simulink model "sg_IK"  (R2021b)
settings: Solver=ode4  StartTime=0.0  StopTime=10  FixedStep=Ts  RelTol=1e-3  EnableMultiTasking=on
model workspace (MAT data in the model file):
  BList = [0 0 -1 0 -2.61918 0 0 1 0 1.41 0 -2.26918 ... (30 elements, 6x5)]
  M = [1 0 0 0 0 1 0 0 0 0 1 0 ... (16 elements, 4x4)]
  Manual_State_Switch = 0
  Operation_Mode = 2
  SList = [0 0 -1 0 0 0 0 1 0 -0.83 0 0.35 ... (30 elements, 6x5)]
  State_Mode_Selector = 2
  Traj_method = 1
  Winch_EnableHeaveComp = 0
  Winch_NewCmd = 0
  Winch_PosRef = 10
  controlMode = 2
  new_command_traj = 0
  v_max = 0
  x_coordinate_traj = 0
  y_coordinate_traj = 0
  z_coordinate_traj = 0
values from neighbouring files (symbols this model uses):
  Ts = 1e-3    (= 0.001)    [sg_IK_build.m]    (also in sg_IK_startup.m)
libraries: slpidlib x5, slrealtimeutilitieslib x3, slrealtimeiplib x3, dspfdesign x1
(part 2 of 2)

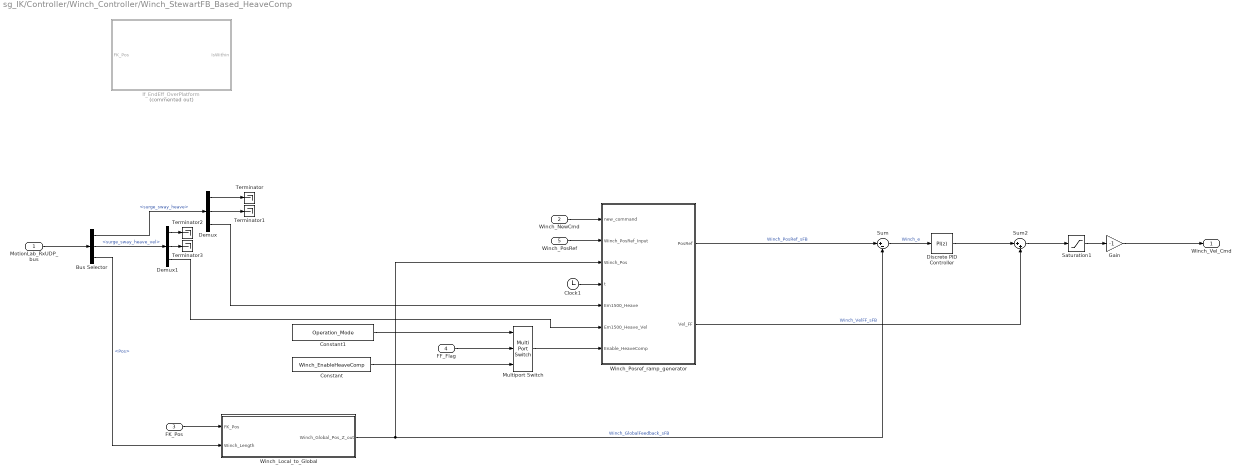
== system sg_IK/Controller/Winch_Controller/Winch_StewartFB_Based_HeaveComp ==
  MotionLab_RxUDP_bus : Inport
  Winch_NewCmd : Inport  Port=2
  FK_Pos : Inport  Port=3
  FF_Flag : Inport  Port=4
  Winch_PosRef : Inport  Port=5
  Bus Selector : BusSelector  OutputSignals=Em1500.surge_sway_heave,Em1500.surge_sway_heave_vel,Comau_winch.Pos
  Clock1 : Clock
  Constant : Constant  Value=Winch_EnableHeaveComp
  Constant1 : Constant  Value=Operation_Mode
  Demux : Demux  Outputs=3
  Demux1 : Demux  Outputs=3
  Discrete PID Controller : slpidlib/PID Controller  Controller=PI  Form=Parallel  TimeDomain=Discrete-time  UseExternalTs=off  SampleTime=Ts  IntegratorMethod=Forward Euler  FilterMethod=Forward Euler  ControllerParametersSource=internal  P=2  I=0.09  D=0  UseFilter=on  N=100  TunerSelectOption=Transfer Function Based (PID Tuner App)  InitialConditionSource=internal  InitialConditionForIntegrator=0  InitialConditionForFilter=0  DifferentiatorICPrevScaledInput=0  ExternalReset=none  TrackingMode=off  Kt=1  LimitOutput=off  SatLimitsSource=internal  UpperSaturationLimit=inf  LowerSaturationLimit=-inf  LinearizeAsGain=off  AntiWindupMode=none  Kb=1  POutMin=[]  POutMax=[]  IOutMin=[]  IOutMax=[]  DOutMin=[]  DOutMax=[]  NOutMin=[]  NOutMax=[]  SumOutMin=[]  SumOutMax=[]  SaturationOutMin=[]  SaturationOutMax=[]  PParamMin=[]  PParamMax=[]  IParamMin=[]  IParamMax=[]  DParamMin=[]  DParamMax=[]  NParamMin=[]  NParamMax=[]  KbParamMin=[]  KbParamMax=[]  KtParamMin=[]  KtParamMax=[]  KbOutMin=[]  KbOutMax=[]  KtOutMin=[]  KtOutMax=[]  IntegratorOutMin=[]  IntegratorOutMax=[]  FilterOutMin=[]  FilterOutMax=[]  SumI1OutMin=[]  SumI1OutMax=[]  SumI2OutMin=[]  SumI2OutMax=[]  SumI3OutMin=[]  SumI3OutMax=[]  SumI4OutMin=[]  SumI4OutMax=[]  SumDOutMin=[]  SumDOutMax=[]  DifferentiatorOutMin=[]  DifferentiatorOutMax=[]  FilterDiffOutCoefMin=[]  FilterDiffOutCoefMax=[]  ReciprocalOutMin=[]  ReciprocalOutMax=[]  SumDenOutMin=[]  SumDenOutMax=[]  SumNumOutMin=[]  SumNumOutMax=[]  DivideOutMin=[]  DivideOutMax=[]  UdiffTsProdOutMin=[]  UdiffTsProdOutMax=[]  NTsProdOutMin=[]  NTsProdOutMax=[]  UintegralTsProdOutMin=[]  UintegralTsProdOutMax=[]  UngainTsProdOutMin=[]  UngainTsProdOutMax=[]  FilterDenConstantOutDataTypeStr=Inherit: Inherit via back propagation  FilterDenConstantOutMin=[]  FilterDenConstantOutMax=[]  PCopyOutDataTypeStr=Inherit: Inherit via back propagation  PCopyOutMin=[]  PCopyOutMax=[]  NCopyOutDataTypeStr=Inherit: Inherit via back propagation  NCopyOutMin=[]  NCopyOutMax=[]  IntegratorContinuousStateAttributes=''  IntegratorStateMustResolveToSignalObject=off  IntegratorRTWStateStorageClass=Auto  FilterContinuousStateAttributes=''  FilterStateMustResolveToSignalObject=off  FilterRTWStateStorageClass=Auto  ParallelPVariant=InternalParameters  IdealPVariant=Disabled  IVariant=InternalParameters  DVariant=Disabled  IntegratorVariant=Discrete  SatVariant=Disabled  AWVariant=Passthrough  PCopyVariant=Disabled  TRVariant=Disabled  FdbkBlocksVariant=Forward  IdealPFdbkVariant=Disabled  SatFdbkVariant=Disabled  DerivativeFilterVariant=Disabled  NVariant=Disabled  NCopyVariant=Disabled_SignalSpec  FilterICVariant=Disabled  IntegratorICVariant=InternalICs  ExternalResetVariant=Disabled  TRSumVariant=Passthrough  SumFdbkVariant=Disabled  SumVariant=Sum_PI  TsampFilterVariant=InternalTs  TsampNgainVariant=Passthrough  TsampIntegralVariant=Passthrough  ExternalSaturationOutDataTypeStr=Inherit: Same as second input
  Gain : Gain  Gain=-1
  If_EndEff_OverPlatform : MATLAB Function  Commented=on  TreatAsAtomicUnit=on
  Multiport Switch : MultiPortSwitch  Inputs=2
  Saturation1 : Saturate  UpperLimit=0.2  LowerLimit=-0.2
  Sum : Sum  Inputs=|+-
  Sum2 : Sum  Inputs=|++
  Terminator{,1..3} (4 alike) : Terminator
  Winch_Local_to_Global : MATLAB Function  TreatAsAtomicUnit=on
  Winch_Posref_ramp_generator : MATLAB Function  TreatAsAtomicUnit=on
  Winch_Vel_Cmd : Outport
  wires:
  Constant/1 -> Multiport Switch/3
  Constant1/1 -> Multiport Switch/1
  Multiport Switch/1 -> Winch_Posref_ramp_generator/7(Enable_HeaveComp)
  Clock1/1 -> Winch_Posref_ramp_generator/4(t)
  Winch_NewCmd/1 -> Winch_Posref_ramp_generator/1(new_command)
  Winch_PosRef/1 -> Winch_Posref_ramp_generator/2(Winch_PosRef_Input)
  FF_Flag/1 -> Multiport Switch/2
  Discrete PID Controller/1 -> Sum2/1
  Winch_Posref_ramp_generator/1(PosRef) -> Sum/1  "Winch_PosRef_sFB"
  Winch_Posref_ramp_generator/2(Vel_FF) -> Sum2/2  "Winch_VelFF_sFB"
  Saturation1/1 -> Gain/1
  Sum/1 -> Discrete PID Controller/1  "Winch_e"
  Sum2/1 -> Saturation1/1
  FK_Pos/1 -> Winch_Local_to_Global/1(FK_Pos)
  MotionLab_RxUDP_bus/1 -> Bus Selector/1
  Bus Selector/3 -> Winch_Local_to_Global/2(Winch_Length)  "<Pos>"
  Winch_Local_to_Global/1(Winch_Global_Pos_Z_out) -> Winch_Posref_ramp_generator/3(Winch_Pos), Sum/2  "Winch_GlobalFeedback_sFB"
  Bus Selector/1 -> Demux/1  "<surge_sway_heave>"
  Demux/1 -> Terminator/1
  Demux/2 -> Terminator1/1
  Demux/3 -> Winch_Posref_ramp_generator/5(Em1500_Heave)
  Bus Selector/2 -> Demux1/1  "<surge_sway_heave_vel>"
  Demux1/1 -> Terminator2/1
  Demux1/2 -> Terminator3/1
  Demux1/3 -> Winch_Posref_ramp_generator/6(Em1500_Heave_Vel)
  Gain/1 -> Winch_Vel_Cmd/1

== matlab function sg_IK/Controller/State Machine and Operation mode selecotr/Winch_Local_to_Global ==
  data: FK_Pos input; Winch_Global_Pos_Z output; Winch_Length input
function Winch_Global_Pos_Z = Winch_Global_Pos(FK_Pos, Winch_Length)
    %constant found from calibrating winch moving it to same height as
    %ball
    vertical_distance = Winch_Length - 0.202; 
    Winch_Global_Pos_Z = FK_Pos(3) - vertical_distance;
end

== matlab function sg_IK/Controller/Winch_Controller/Winch_StewartFB_Based_HeaveComp/Winch_Local_to_Global ==
  data: FK_Pos input; Winch_Global_Pos_Z_out output; Winch_Length input
function Winch_Global_Pos_Z_out = Winch_Global_Pos( FK_Pos, Winch_Length)

vertical_distance = Winch_Length - 0.202; 

Winch_Global_Pos_Z_out = FK_Pos(3) - vertical_distance;



end

== matlab function sg_IK/Controller/State Machine and Operation mode selecotr/is_Em8000_settled ==
  data: Em8000_translation input; Em8000_settled_flag output
function Em8000_settled_flag = settled_fnc(Em8000_translation)
Em8000_heave = Em8000_translation(3);

%Flag for if platform is in settled position
%More better handling would be a direct feedback from the Em1500 IPC what operation mode the platform is in
if Em8000_heave >= 0.99 && Em8000_heave <= 1.01 %Em1500 platform is in settled mode
    Em8000_settled_flag = true;
else
    Em8000_settled_flag = false;
end

== stateflow chart sg_IK/Controller/State Machine and Operation mode selecotr/Chart ==
  state Manual_State_Switch_Mode
    state Go_home
      entry:
      if Em8000_settled_flag && ~Em8000_comp_offset_flag
      Em8000_settled_offset = 1;
      elseif Em8000_comp_offset_flag
      Em8000_settled_offset = 0.65;
      else
      Em8000_settled_offset = 0;
      end
      X_home = -0.9;
      Y_home = -1.3;
      Z_home = 5.9 - Em8000_settled_offset;
      Traj_points_XYZ = [FK_Pos(1), X_home, FK_Pos(2), Y_home, FK_Pos(3), Z_home];
      Traj_method = 2;
      v_max = 0.1;
      new_command = new_command + 1;
      Winch_PosRef = 10; %JUST MOVE UP, MAKE MORE ROBUST LATER
      Winch_Mode_selector = 1;
      FF_Flag = 0;
    state Stay_in_current_position
      entry:
      % Set the values for the variables
      Traj_points_XYZ = [FK_Pos(1), FK_Pos(1), FK_Pos(2), FK_Pos(2), FK_Pos(3), FK_Pos(3)];
      Traj_method = 1;
      v_max = 0;
      new_command = new_command + 1;
      FF_Flag = 0;
      Winch_PosRef = 10; %Just move up to endstop
      Winch_Mode_selector = 1; %REMOVE LATER
    state Move_to_above_platform_PickUp
      %Move above platform to initiate hooking and pick up of payload
      entry:
      if Em8000_settled_flag && ~Em8000_comp_offset_flag
      Em8000_settled_offset = 1;
      elseif Em8000_comp_offset_flag
      Em8000_settled_offset = 0.65;
      else
      Em8000_settled_offset = 0;
      end
      X_Platform = 0.42;
      Y_Platform = -1.57;
      Z_Platform = 5.62 - Em8000_settled_offset;
      Traj_points_XYZ = [FK_Pos(1), X_Platform, FK_Pos(2), Y_Platform, FK_Pos(3), Z_Platform];
      Traj_method = 2;
      v_max = 0.12;
      new_command = new_command + 1;
      %move winch
      Winch_Mode_selector = 1;
      Winch_PosRef = 3.2;
      %Winch_NewCmd = Winch_NewCmd + 1;
      FF_Flag = 0;
      during:
      Winch_PosRef = 3.2;
    state Hook_Ball
      state Ball_In_Frame
        %If ball not in frame wait over platform
        entry:
        if bBall_InFrame
        Sub_stage_switch = 1;
        else
        Sub_stage_switch = 0;
        Traj_points_XYZ = [FK_Pos(1), FK_Pos(1), FK_Pos(2), FK_Pos(2), FK_Pos(3), FK_Pos(3)];
        v_max = 0;
        new_command = new_command + 1;
        end
        during:
        if bBall_InFrame
        Sub_stage_switch = 1;
        end
      state Move_Close_To_Ball
        entry:
        Z_Offset = 0.15;
        r_Offset = 0.15;  % Radius offset to ball
        % Compute the approach vector in xy plane
        delta_xy = FK_Pos(1:2) - Ball_Pos(1:2);
        norm_delta = norm(delta_xy);
        if norm_delta < 1e-6
        Target_Pos_X = FK_Pos(1);
        Target_Pos_Y = FK_Pos(2);
        v_max = 0;
        else
        unit_delta = delta_xy / norm_delta;
        Target_Pos_X = Ball_Pos(1) + r_Offset * unit_delta(1);
        Target_Pos_Y = Ball_Pos(2) + r_Offset * unit_delta(2);
        v_max = 0.05;
        end
        %Target_Pos_Z = Ball_Pos(3) + Winch_PosRef + Z_Offset;
        Traj_points_XYZ = [FK_Pos(1), Target_Pos_X, FK_Pos(2), Target_Pos_Y, FK_Pos(3), FK_Pos(3)];
        Traj_method = 2;
        new_command = new_command + 1;
        Winch_PosRef = Ball_Pos(3) - Z_Offset;
        FF_Flag = 1;
        during:
        Winch_PosRef = Ball_Pos(3) - Z_Offset;
        if ~traj_running
        Sub_stage_switch = 2;
        else
        Sub_stage_switch = 1;
        end
      state Move_in_to_ball
        entry:
        Z_Offset = 0.07;
        %Winch_neutral_length = Winch_PosRef;
        Traj_points_XYZ = [FK_Pos(1), Ball_Pos(1), FK_Pos(2), Ball_Pos(2)+0.04, FK_Pos(3), FK_Pos(3)];
        Traj_method = 2;
        v_max = 0.02;
        new_command = new_command + 1;
        Winch_PosRef = Ball_Pos(3);
        FF_Flag = 1;
        during:
        %CB_Absdelta_X = abs(Ball_Pos(1) - Claw_Pos(1));
        %CB_Absdelta_Y = abs(Ball_Pos(2) - Claw_Pos(2));
        Winch_PosRef = Ball_Pos(3) - Z_Offset;
        if ~traj_running
        Sub_stage_switch = 3;
        else
        Sub_stage_switch = 2;
        end
      state Lift_Up
        entry:
        FF_Flag = 0;
        Winch_PosRef = 10;
      (default) -> Manual_State_Switch_Mode.Hook_Ball.Ball_In_Frame
      Manual_State_Switch_Mode.Hook_Ball.Ball_In_Frame -> Manual_State_Switch_Mode.Hook_Ball.Move_Close_To_Ball : [Sub_stage_switch == 1]
      Manual_State_Switch_Mode.Hook_Ball.Move_Close_To_Ball -> Manual_State_Switch_Mode.Hook_Ball.Move_in_to_ball : [Sub_stage_switch == 2 && after(1, sec)]
      Manual_State_Switch_Mode.Hook_Ball.Move_in_to_ball -> Lift_Up : [Sub_stage_switch == 3]
    state Lower_payload_Onto_platform
      state Move_above_platform_While_lowering_payload
        %Move above platform and start moving winch down to stewart platform netrual position to follow
        %And follow heave motion
        entry:
        if Em8000_settled_flag && ~Em8000_comp_offset_flag
        Em8000_settled_offset = 1;
        elseif Em8000_comp_offset_flag
        Em8000_settled_offset = 0.65;
        else
        Em8000_settled_offset = 0;
        end
        Sub_stage_switch2 = 0;
        X_Platform = 0.41;
        Y_Platform = -1.34;
        Z_Platform = 5.67 - Em8000_settled_offset;
        Traj_points_XYZ = [FK_Pos(1), X_Platform, FK_Pos(2), Y_Platform, FK_Pos(3), Z_Platform];
        Traj_method = 2;
        v_max = 0.12;
        new_command = new_command + 1;
        %move winch
        Winch_Mode_selector = 2;
        Winch_PosRef = 2.6;
        Winch_NewCmd = Winch_NewCmd + 1;
        FF_Flag = 1;
        during:
        if ~traj_running
        Sub_stage_switch2 = 1;
        end
      state Lower_winch_To_unhook
        entry:
        Winch_PosRef = 2.6;
        Winch_NewCmd = Winch_NewCmd + 1;
      state Move_to_side_unhook
        entry:
        if Em8000_settled_flag && ~Em8000_comp_offset_flag
        Em8000_settled_offset = 1;
        elseif Em8000_comp_offset_flag
        Em8000_settled_offset = 0.65;
        else
        Em8000_settled_offset = 0;
        end
        X_Unhook = 0;
        Y_Unhook = -1.62;
        Z_Unhook = 5.62 - Em8000_settled_offset;
        Traj_points_XYZ = [FK_Pos(1), X_Unhook, FK_Pos(2), Y_Unhook, FK_Pos(3), Z_Unhook];
        Traj_method = 2;
        v_max = 0.07;
        new_command = new_command + 1;
        %move winch
        Winch_PosRef = 2.6;
        Winch_NewCmd = Winch_NewCmd + 1;
        FF_Flag = 1;
      (default) -> Manual_State_Switch_Mode.Lower_payload_Onto_platform.Move_above_platform_While_lowering_payload
      Manual_State_Switch_Mode.Lower_payload_Onto_platform.Move_above_platform_While_lowering_payload -> Manual_State_Switch_Mode.Lower_payload_Onto_platform.Lower_winch_To_unhook : [Sub_stage_switch2 == 1 && after(3, sec)]
      Manual_State_Switch_Mode.Lower_payload_Onto_platform.Lower_winch_To_unhook -> Manual_State_Switch_Mode.Lower_payload_Onto_platform.Move_to_side_unhook : [after(7, sec)]
    (default) -> Stay_in_current_position
    Manual_State_Switch_Mode.Lower_payload_Onto_platform -> Manual_State_Switch_Mode.Go_home [order 1] : [Switch == 1]
    Manual_State_Switch_Mode.Go_home -> Manual_State_Switch_Mode.Lower_payload_Onto_platform [order 3] : [Switch == 4]
    Stay_in_current_position -> Manual_State_Switch_Mode.Go_home [order 1] : [Switch == 1]
    Manual_State_Switch_Mode.Hook_Ball -> Manual_State_Switch_Mode.Go_home [order 2] : [Switch == 1]
    Manual_State_Switch_Mode.Go_home -> Stay_in_current_position [order 1] : [Switch == 0]
    Manual_State_Switch_Mode.Lower_payload_Onto_platform -> Stay_in_current_position [order 2] : [Switch == 0]
    Manual_State_Switch_Mode.Hook_Ball -> Stay_in_current_position [order 3] : [Switch == 0]
    Manual_State_Switch_Mode.Move_to_above_platform_PickUp -> Stay_in_current_position [order 1] : [Switch == 0]
    Stay_in_current_position -> Manual_State_Switch_Mode.Move_to_above_platform_PickUp [order 2] : [Switch == 2]
    Manual_State_Switch_Mode.Move_to_above_platform_PickUp -> Manual_State_Switch_Mode.Go_home [order 2] : [Switch == 1]
    Manual_State_Switch_Mode.Go_home -> Manual_State_Switch_Mode.Move_to_above_platform_PickUp [order 2] : [Switch == 2]
    Manual_State_Switch_Mode.Move_to_above_platform_PickUp -> Manual_State_Switch_Mode.Hook_Ball [order 3] : [Switch == 3]
    Manual_State_Switch_Mode.Hook_Ball -> Manual_State_Switch_Mode.Move_to_above_platform_PickUp [order 1] : [Switch==2]
  state Mode_selector_state
    entry:
    %Entry state to choose between manual state switch mode or Autonomous mode
    if State_Mode_Selector == 1 %Autonomous mode
    Hook_state_switch = 1;
    Mode = 1;
    elseif  State_Mode_Selector == 2 %Manual state switch mode
    Mode = 2;
    else %Default to Manual state switch mode
    Mode = 2;
    end
  state Autonomous_Operation_Mode
    state Go_home
      entry:
      AutoSwitch = 0;
      if Em8000_settled_flag && ~Em8000_comp_offset_flag
      Em8000_settled_offset = 1;
      elseif Em8000_comp_offset_flag
      Em8000_settled_offset = 0.65;
      else
      Em8000_settled_offset = 0;
      end
      X_home = -0.9;
      Y_home = -1.3;
      Z_home = 5.9 - Em8000_settled_offset;
      Traj_points_XYZ = [FK_Pos(1), X_home, FK_Pos(2), Y_home, FK_Pos(3), Z_home];
      Traj_method = 2;
      v_max = 0.1;
      new_command = new_command + 1;
      Winch_PosRef = 10; %JUST MOVE UP, MAKE MORE ROBUST LATER
      Winch_Mode_selector = 1;
      FF_Flag = 0;
      during:
      if ~traj_running
      if Hook_state_switch == 1
      AutoSwitch = 1; %Hook payload
      else
      AutoSwitch = 2; %Lower payload
      end
      else
      AutoSwitch = 0; %Stay in current state until traj to home complete
      end
    state Hook_Ball
      state Move_to_above_platform_PickUp
        %Move above platform to initiate hooking and pick up of payload
        entry:
        if Em8000_settled_flag && ~Em8000_comp_offset_flag
        Em8000_settled_offset = 1;
        elseif Em8000_comp_offset_flag
        Em8000_settled_offset = 0.65;
        else
        Em8000_settled_offset = 0;
        end
        X_Platform = 0.42;
        Y_Platform = -1.57;
        Z_Platform = 5.62 - Em8000_settled_offset;
        Traj_points_XYZ = [FK_Pos(1), X_Platform, FK_Pos(2), Y_Platform, FK_Pos(3), Z_Platform];
        Traj_method = 2;
        v_max = 0.16;
        new_command = new_command + 1;
        %move winch
        Winch_Mode_selector = 1;
        Winch_PosRef = 3.15;
        %Winch_NewCmd = Winch_NewCmd + 1;
        FF_Flag = 1;
        during:
        Winch_PosRef = 3.15;
        if ~traj_running
        Sub_stage_switch = 1;
        end
      state Ball_In_Frame
        %If ball not in frame wait over platform
        entry:
        if bBall_InFrame
        Sub_stage_switch = 1;
        else
        Sub_stage_switch = 0;
        Traj_points_XYZ = [FK_Pos(1), FK_Pos(1), FK_Pos(2), FK_Pos(2), FK_Pos(3), FK_Pos(3)];
        v_max = 0;
        new_command = new_command + 1;
        end
        during:
        if bBall_InFrame
        Sub_stage_switch = 2;
        else
        Sub_stage_switch = 1;
        end
      state Move_Close_To_Ball
        entry:
        Z_Offset = 0.15;
        r_Offset = 0.15;  % Radius offset to ball
        % Compute the approach vector in xy plane
        delta_xy = FK_Pos(1:2) - Ball_Pos(1:2);
        norm_delta = norm(delta_xy);
        if norm_delta < 1e-6
        Target_Pos_X = FK_Pos(1);
        Target_Pos_Y = FK_Pos(2);
        v_max = 0;
        else
        unit_delta = delta_xy / norm_delta;
        Target_Pos_X = Ball_Pos(1) + r_Offset * unit_delta(1);
        Target_Pos_Y = Ball_Pos(2) + r_Offset * unit_delta(2);
        v_max = 0.02;
        end
        %Target_Pos_Z = Ball_Pos(3) + Winch_PosRef + Z_Offset;
        Traj_points_XYZ = [FK_Pos(1), Target_Pos_X, FK_Pos(2), Target_Pos_Y, FK_Pos(3), FK_Pos(3)];
        Traj_method = 2;
        new_command = new_command + 1;
        Winch_PosRef = Ball_Pos(3) - Z_Offset;
        FF_Flag = 1;
        during:
        Winch_PosRef = Ball_Pos(3) - Z_Offset;
        if ~traj_running
        Sub_stage_switch = 3;
        else
        Sub_stage_switch = 2;
        end
      state Move_in_to_ball
        entry:
        Z_Offset = 0.07;
        %Winch_neutral_length = Winch_PosRef;
        Traj_points_XYZ = [FK_Pos(1), Ball_Pos(1), FK_Pos(2), Ball_Pos(2)+0.06, FK_Pos(3), FK_Pos(3)];
        Traj_method = 2;
        v_max = 0.02;
        new_command = new_command + 1;
        Winch_PosRef = Ball_Pos(3);
        FF_Flag = 1;
        during:
        %CB_Absdelta_X = abs(Ball_Pos(1) - Claw_Pos(1));
        %CB_Absdelta_Y = abs(Ball_Pos(2) - Claw_Pos(2));
        Winch_PosRef = Ball_Pos(3) - Z_Offset;
        if ~traj_running
        AutoSwitch = 0;
        else
        Sub_stage_switch = 2;
        end
        exit:
        Sub_stage_switch = 0;
        Hook_state_switch = 0; %Payload was picked up mark next exit from Go_to_home to lower payload
      (default) -> Autonomous_Operation_Mode.Hook_Ball.Move_to_above_platform_PickUp
      Autonomous_Operation_Mode.Hook_Ball.Move_to_above_platform_PickUp -> Autonomous_Operation_Mode.Hook_Ball.Ball_In_Frame : [Sub_stage_switch == 1 && after(1, sec)]
      Autonomous_Operation_Mode.Hook_Ball.Ball_In_Frame -> Autonomous_Operation_Mode.Hook_Ball.Move_Close_To_Ball : [Sub_stage_switch == 2]
      Autonomous_Operation_Mode.Hook_Ball.Move_Close_To_Ball -> Autonomous_Operation_Mode.Hook_Ball.Move_in_to_ball : [Sub_stage_switch == 3 && after(0.5, sec)]
    state Lower_payload_Onto_platform
      state Move_above_platform_While_lowering_payload
        %Move above platform and start moving winch down to stewart platform netrual position to follow
        %And follow heave motion
        entry:
        if Em8000_settled_flag && ~Em8000_comp_offset_flag
        Em8000_settled_offset = 1;
        elseif Em8000_comp_offset_flag
        Em8000_settled_offset = 0.65;
        else
        Em8000_settled_offset = 0;
        end
        Sub_stage_switch2 = 0;
        X_Platform = 0.41;
        Y_Platform = -1.34;
        Z_Platform = 5.67 - Em8000_settled_offset;
        Traj_points_XYZ = [FK_Pos(1), X_Platform, FK_Pos(2), Y_Platform, FK_Pos(3), Z_Platform];
        Traj_method = 2;
        v_max = 0.16;
        new_command = new_command + 1;
        %move winch
        Winch_Mode_selector = 2;
        Winch_PosRef = 3.2;
        Winch_NewCmd = Winch_NewCmd + 1;
        FF_Flag = 1;
        during:
        if ~traj_running
        Sub_stage_switch2 = 1;
        end
      state Lower_winch_To_unhook
        entry:
        Winch_PosRef = 3.04;
        Winch_NewCmd = Winch_NewCmd + 1;
      state Move_to_side_unhook
        entry:
        if Em8000_settled_flag && ~Em8000_comp_offset_flag
        Em8000_settled_offset = 1;
        elseif Em8000_comp_offset_flag
        Em8000_settled_offset = 0.65;
        else
        Em8000_settled_offset = 0;
        end
        X_Unhook = 0;
        Y_Unhook = -1.62;
        Z_Unhook = 5.62 - Em8000_settled_offset;
        Traj_points_XYZ = [FK_Pos(1), X_Unhook, FK_Pos(2), Y_Unhook, FK_Pos(3), Z_Unhook];
        Traj_method = 2;
        v_max = 0.07;
        new_command = new_command + 1;
        %move winch
        Winch_PosRef = 3.01;
        Winch_NewCmd = Winch_NewCmd + 1;
        FF_Flag = 1;
        during:
        if ~traj_running
        AutoSwitch = 0;
        end
        exit:
        Sub_stage_switch2 = 0;
        Hook_state_switch = 1; %Payload was lowered down mark next exit from Go_to_home to pickup payload
      (default) -> Autonomous_Operation_Mode.Lower_payload_Onto_platform.Move_above_platform_While_lowering_payload
      Autonomous_Operation_Mode.Lower_payload_Onto_platform.Move_above_platform_While_lowering_payload -> Autonomous_Operation_Mode.Lower_payload_Onto_platform.Lower_winch_To_unhook : [Sub_stage_switch2 == 1 && after(1, sec)]
      Autonomous_Operation_Mode.Lower_payload_Onto_platform.Lower_winch_To_unhook -> Autonomous_Operation_Mode.Lower_payload_Onto_platform.Move_to_side_unhook : [after(5, sec)]
    (default) -> Autonomous_Operation_Mode.Go_home
    Autonomous_Operation_Mode.Lower_payload_Onto_platform -> Autonomous_Operation_Mode.Go_home : [AutoSwitch == 0 && after(1, sec)]
    Autonomous_Operation_Mode.Go_home -> Autonomous_Operation_Mode.Lower_payload_Onto_platform [order 2] : [AutoSwitch == 2 && after(3, sec)]
    Autonomous_Operation_Mode.Hook_Ball -> Autonomous_Operation_Mode.Go_home : [AutoSwitch == 0 && after(1, sec)]
    Autonomous_Operation_Mode.Go_home -> Autonomous_Operation_Mode.Hook_Ball [order 1] : [AutoSwitch == 1 && after(3, sec)]
  (default) -> Mode_selector_state
  Mode_selector_state -> Manual_State_Switch_Mode [order 1] : [Mode == 2]
  Mode_selector_state -> Autonomous_Operation_Mode [order 2] : [Mode == 1]
  data: State_Mode_Selector input; Switch input; Em8000_comp_offset_flag input; Traj_points_XYZ output; new_command output =0; Traj_method output; v_max output =0; FK_Pos input; Claw_Pos input; bBall_InFrame input; Em8000_settled_flag input; Z_home local; X_home local; Y_home local; X_Platform local; Z_Platform local; Y_Platform local; Ball_Pos input; Winch_Pos_world input; Z_Offset local; r_Offset local; Target_Pos_Y local; Target_Pos_X local; Target_Pos_Z local; unit_delta local; Sub_stage_switch local; traj_running input; Z_Up local; norm_delta local; delta_xy local; Winch_NewCmd output =0; Winch_PosRef output; Winch_Mode_selector output; FF_Flag output; Mode local; Sub_stage_switch2 local; X_Unhook local; Y_Unhook local; Z_Unhook local; Em8000_settled_offset local; Hook_state_switch local; AutoSwitch local

== matlab function sg_IK/Controller/Inverse velocity and forward kinematics/Forward kinematics/FK_solver ==
  data: thetalist input; Endeff_local_xyz output; T_w_ee output; M input; SList input; Em8000_RPY input; Em8000_tr input; T_b_ee output; Endeff_world_xyz output
function [Endeff_local_xyz, T_w_ee, T_b_ee, Endeff_world_xyz]  = FK_cartPos(thetalist, M, SList, Em8000_RPY, Em8000_tr)
%Compute end effector frame from Forward kinematics to measure end effector
%position
T_b_ee = FKinSpace(M,SList,thetalist); %Keep in local robot base frame coordinates for IK solver

cartPos = [T_b_ee(1:3,4)];

Endeff_local_xyz = cartPos;

%% Transform to world frame for trajectory planner 
Em8000_RPY = [Em8000_RPY(1) Em8000_RPY(2) Em8000_RPY(3)];

%From world frame to platform frame
w_s_quat = [6.0198987883e-05, 0.705931944115, 0.708279565403954, 0.000379322138596];

R_w_p = quat2rotm(w_s_quat);
tr_w_p = [-2.969661622702265, 1.976311036084776, 2.662845015592614]';


%platform frame to comau
p_c_quat = [0.002461288106714, -0.501408337431486, -0.865206982556575, 0.000706081011787];

R_p_c = quat2rotm(p_c_quat); %rotation matrix
tr_p_c = [-1.082024099747949, 1.536041691521612, -1.024461448780775]'; %Translational vector


R_pBody = eul2rotm(Em8000_RPY,"XYZ"); %Dynamic rotation of the platform body 

T_w_p_static = [R_w_p, tr_w_p; zeros(1,3), 1]; %Static transform from EM8000 platform to world frame

T_pBody = [R_pBody, Em8000_tr; zeros(1,3), 1]; %Transformation matrix of the dynamic movement of the platform (rotation and translation seen from the origon of the platform ie not in world frame)

T_w_p = T_w_p_static * T_pBody; %Transform from world frame to moving platform frame

T_p_c_static = [R_p_c, tr_p_c; zeros(1,3), 1]; %Static transformation between platform frame and comau robot base frame

T_w_c = T_w_p * T_p_c_static;

T_w_ee = T_w_c * T_b_ee;

Endeff_world_xyz = [T_w_ee(1:3,4)];

== matlab function sg_IK/Controller/Inverse velocity and forward kinematics/IVK_solver ==
  data: thetaListDot output size=[5, 1]; Em8000_tr input; Em8000_vel input; Em8000_omega input; Em8000_RPY input; T_b_ee input; Traj_vel input; thetaList0 input; BList input; Ts input; Joint_LimitReached output boolean size=[1 1]; q_measured input
function [thetaListDot, Joint_LimitReached] = inverseKinematics( ...
    Em8000_tr, Em8000_vel, Em8000_omega, Em8000_RPY, T_b_ee, Traj_vel, thetaList0, BList, Ts, q_measured)



Em8000_RPY = [Em8000_RPY(1) Em8000_RPY(2) Em8000_RPY(3)];

%From world frame to platform frame
w_p_quat = [6.0198987883e-05, 0.705931944115, 0.708279565403954, 0.000379322138596];
R_w_p    = quat2rotm(w_p_quat);
tr_w_p   = [-2.969661622702265, 1.976311036084776, 3.312845015592614]';

%platform frame to comau
p_c_quat = [0.002461288106714, -0.501408337431486, -0.865206982556575, 0.000706081011787];
R_p_c    = quat2rotm(p_c_quat); %rotation matrix
tr_p_c   = [-1.082024099747949, 1.536041691521612, -0.3]'; %Translational vector

R_pBody      = eul2rotm(Em8000_RPY,"XYZ"); %Dynamic rotation of the platform body 
T_w_p_static = [R_w_p,    tr_w_p;    zeros(1,3), 1]; %Static transform from EM8000 platform to world frame
T_pBody      = [R_pBody, Em8000_tr; zeros(1,3), 1];  %Transformation matrix of the dynamic movement of the platform
T_w_p        = T_w_p_static * T_pBody;               %Transform from world frame to moving platform frame

T_p_c_static = [R_p_c,    tr_p_c;    zeros(1,3), 1]; %Static transformation between platform frame and comau robot base frame
T_w_c        = T_w_p * T_p_c_static;
T_w_ee       = T_w_c * T_b_ee;



Jb      = JacobianBody(BList, thetaList0);
Jb_pinv = pinv(Jb);

%Desired end effector twist vector of trajectory
V_traj_world = [0; 0; 0; Traj_vel(1); Traj_vel(2); Traj_vel(3)];

%Twist vector of platform motion
V_p        = [Em8000_omega(1); Em8000_omega(2); Em8000_omega(3);
              Em8000_vel(1);   Em8000_vel(2);   Em8000_vel(3)];

%Twist vector of platform expressed in world frame
V_p_world  = Adjoint(T_w_p) * V_p;

%Twist vector of platform expressed in dynamic robot end effector frame
V_p_ee = Adjoint(TransInv(T_w_ee)) * V_p_world;

%Twist vector of trajectory expressed in dynamic robot end effector frame
V_traj_ee = Adjoint(TransInv(T_w_ee)) * V_traj_world;

%Inverse velocity kinematics mr chapter 6.3
thetaListDot = Jb_pinv * (V_traj_ee - V_p_ee);

%Joint limits
q1_LowerLimit = -90;   q2_LowerLimit = -45;  q3_LowerLimit = -110;
q1_UpperLimit =  95;   q2_UpperLimit =  30;  q3_UpperLimit =  -45;
lower_limits  = [q1_LowerLimit;  q2_LowerLimit;  q3_LowerLimit] * pi/180;
upper_limits  = [q1_UpperLimit;  q2_UpperLimit;  q3_UpperLimit] * pi/180;

theta_predicted = q_measured + thetaListDot(1:3) * Ts;

if any(theta_predicted < lower_limits) || any(theta_predicted > upper_limits)
    %Joint limit reached and safe mode engaded
    thetaListDot      = zeros(size(thetaListDot));
    Joint_LimitReached = true;
else
    Joint_LimitReached = false;
end

end

== matlab function sg_IK/Controller/Trajectory planner/Trajectory_planner ==
  data: points_x input size=[1 2]; points_y input size=[1 2]; points_z input size=[1 2]; p output double size=[1 3]; t input size=[1 1]; p_vel output double size=[1 3]; new_command input size=[1 1]; Traj_Running output boolean size=[1 1]; traj_method input size=[1 1]; v_max input size=[1 1]; Joint_limitFlag input boolean size=[1 1]
function [p, p_vel, Traj_Running] = TrajectoryGen(points_x, points_y, points_z, t, new_command, traj_method, v_max, Joint_limitFlag)
%#codegen

p     = zeros(1, 3);
p_vel = zeros(1, 3);

%If a joint limit violation is detected, hold the current position and exit function until
%system reset for safety
if Joint_limitFlag
    p     = [points_x(1), points_y(1), points_z(1)];
    p_vel = [0, 0, 0];
    Traj_Running = false;
    return;
end

%Persistent variables for timing, command tracking, and to hold new
%trajectory points
persistent abs_tf base_t last_command 
persistent new_points_x new_points_y new_points_z

if isempty(abs_tf)
  abs_tf       = 0;
  base_t       = 0;
  last_command = 0;
  new_points_x = points_x;
  new_points_y = points_y;
  new_points_z = points_z;
end

%New command detected counted up
if new_command ~= last_command
    %Capture the current time as the start time
    base_t = t;
  
    new_points_x = points_x;
    new_points_y = points_y;
    new_points_z = points_z;
    
    %Calculate trajectory duration T based on Vmax
    %Ensure Vmax is not too small and avoid division by zero
    T_min = 1e-6;
    v_max = max(v_max, T_min);
    
    %Estimate trajectory time based on a max velocity
    T_x = abs(new_points_x(2) - new_points_x(1)) / v_max;
    T_y = abs(new_points_y(2) - new_points_y(1)) / v_max;
    T_z = abs(new_points_z(2) - new_points_z(1)) / v_max;
    
    %Choose the maximum time required among all three axes to synchronize
    %trajecory 
    T = max([T_x, T_y, T_z, T_min]);
    
    %Set the absolute finish time based on the computed duration
    abs_tf = T + t;
    
    last_command = new_command;
end

%local time variables for trajectory
local_t  = t - base_t;
local_tf = abs_tf - base_t;


if abs_tf == 0  || v_max == 0 %Trajectory not initialized or v_max = 0 hold current position
    x_pos = new_points_x(1);
    y_pos = new_points_y(1);
    z_pos = new_points_z(1);
    
    x_vel = 0;
    y_vel = 0;
    z_vel = 0;
else
    if traj_method == 1 %Cubic trajectory
        [x_pos, x_vel, ~] = cubicTrajectoryPlanner(local_t, local_tf, new_points_x(1), new_points_x(2), 0, 0);
        [y_pos, y_vel, ~] = cubicTrajectoryPlanner(local_t, local_tf, new_points_y(1), new_points_y(2), 0, 0);
        [z_pos, z_vel, ~] = cubicTrajectoryPlanner(local_t, local_tf, new_points_z(1), new_points_z(2), 0, 0);
    elseif traj_method == 2 %Quintic trajectory
        [x_pos, x_vel, ~] = quinticTrajectoryPlanner(local_t, local_tf, new_points_x(1), new_points_x(2), 0, 0, 0, 0);
        [y_pos, y_vel, ~] = quinticTrajectoryPlanner(local_t, local_tf, new_points_y(1), new_points_y(2), 0, 0, 0, 0);
        [z_pos, z_vel, ~] = quinticTrajectoryPlanner(local_t, local_tf, new_points_z(1), new_points_z(2), 0, 0, 0, 0);
    else %Default cubic
        [x_pos, x_vel, ~] = cubicTrajectoryPlanner(local_t, local_tf, new_points_x(1), new_points_x(2), 0, 0);
        [y_pos, y_vel, ~] = cubicTrajectoryPlanner(local_t, local_tf, new_points_y(1), new_points_y(2), 0, 0);
        [z_pos, z_vel, ~] = cubicTrajectoryPlanner(local_t, local_tf, new_points_z(1), new_points_z(2), 0, 0);
    end
end

% local_tf_log = local_tf;
% local_t_log = local_t;


p(1)     = x_pos;
p(2)     = y_pos;
p(3)     = z_pos;

p_vel(1) = x_vel;
p_vel(2) = y_vel;
p_vel(3) = z_vel;

Traj_Running = (t <= abs_tf + 0.1); %Trajectory complete flag with 0.1 second buffer
end

== matlab function sg_IK/Controller/UDP_Camera/Camera_transform ==
  data: p_cam input; p_Ball_space output; p_Claw_space output; T_w_ee input; Camera_IMU_Quart input; Camera_space_frame_XYZ output; Camera_space_frame_EUL output; bBall_InFrame output
function [p_Ball_space, p_Claw_space, Camera_space_frame_XYZ, Camera_space_frame_EUL, bBall_InFrame] = transformFrame(p_cam, T_w_ee, Camera_IMU_Quart)
%Extract ball and claw position vectors in the camera local frame
p_Ball_camera = p_cam(1:3);
p_Claw_camera = p_cam(4:6);

%Reorder quaternion from luxonis [x; y; z; w] to MATLAB quat [w, x, y, z]
q = [Camera_IMU_Quart(4), Camera_IMU_Quart(1), Camera_IMU_Quart(2), Camera_IMU_Quart(3)];

%Camera imu is inacurate aligning it with local frame by adding raw
%measurements from imu when camera is pointing down at rest
q_offset = [0 0.0160522 0.080932 0.0632324];
q = q + q_offset;
%q = [1 0 0 0];
R_cam = quat2rotm(q);

%Static translation from end effector to camera
%t_ee_c = [0.08; -0.08; -0.50];
%t_ee_c = [0.02; -0.21; -0.50];
t_ee_c = [-0.10; -0.03; -0.50]; %[-0.15; -0.12; -0.50];

%Transformation frame form end effector to camera
T_ee_c = [R_cam, t_ee_c; 0 0 0 1];

%FK_pos cartesian end effector position expressed in the world frame
%Rotation of robot base frame about space Z axis


t_w_ee = T_w_ee(1:3,4);
%Extract yaw rotation from T_w_ee
R_full  = T_w_ee(1:3,1:3);
yaw     = atan2( R_full(2,1), ...
                 R_full(1,1) );
R_z     = [ cos(yaw) -sin(yaw) 0; 
            sin(yaw)  cos(yaw) 0; 
              0         0      1 ];
%T_w_ee with only yaw rotation
T_w_ee_simp = [ R_z,   t_w_ee; 
                0 0 0    1    ];

%Transformation from world frame to camera frame
T_w_c = T_w_ee_simp * T_ee_c;

%Extract camera position and euler angles in the world frame
Camera_space_frame_XYZ = T_w_c(1:3,4);
Camera_space_frame_R = T_w_c(1:3,1:3);
Camera_space_frame_EUL = rotm2eul(Camera_space_frame_R, 'XYZ');

%Transform ball and claw position measurements from the camera frame to the Base Frame
%T_offset rotates camera measurments to correct orientation
R_offset = roty(-pi) * rotz(-pi/2);
T_offset = [R_offset, zeros(3,1); 0 0 0 1];

%Transformation matrix of measurements with offset rotation
p_Ball_hom = T_offset * [p_Ball_camera; 1];
p_Claw_hom = T_offset * [p_Claw_camera; 1];

%Transform camera measurments to world (space) frame
p_Ball_trans = T_w_c * p_Ball_hom;
p_Claw_trans = T_w_c * p_Claw_hom;
p_Ball_space = p_Ball_trans(1:3);
p_Claw_space = p_Claw_trans(1:3);

%Ball and claw out of frame flag
persistent p_Ball_space_persistent p_Claw_space_persistent;
if isempty(p_Ball_space_persistent)
    p_Ball_space_persistent = p_Ball_space;
end
if isempty(p_Claw_space_persistent)
    p_Claw_space_persistent = p_Claw_space;
end

%Check if ball and claw are within reasonable measurements if completely
%Raw measurments out of frame +-32.8m
bBall_InFrame = true;
bClawInFrame = true;
for i = 1:3
    if (abs(p_Ball_camera(i)) >= 20.0) || (abs(p_Ball_camera(i)) <= -5)
        bBall_InFrame = false;
    end
    if (abs(p_Claw_camera(i)) >= 20.0) || (abs(p_Claw_camera(i)) <= -5)
        bClawInFrame = false;
    end
end
%Hold last known ball and claw position in world frame if ball or claw out
%of camera view
if bBall_InFrame
    p_Ball_space_persistent = p_Ball_space;
else
    p_Ball_space = p_Ball_space_persistent;
end

if bClawInFrame
    p_Claw_space_persistent = p_Claw_space;
else
    p_Claw_space = p_Claw_space_persistent;
end

end

%% standard matlab functions didnt work as expected for some reason
function R = roty(theta)
    R = [ cos(theta)  0 sin(theta);
          0           1 0;
         -sin(theta)  0 cos(theta)];
end

function R = rotz(theta)
    R = [cos(theta) -sin(theta) 0;
         sin(theta)  cos(theta) 0;
         0           0          1];
end

== matlab function sg_IK/Controller/Winch_Controller/Winch_Camera_Based_HeaveComp/FeedForward_Switch ==
  data: Stewart_Heave_Vel input; Vel_FF output; FF_Flag input
function Vel_FF = fcn(Stewart_Heave_Vel, FF_Flag)
    FF_Flag = logical(FF_Flag);
    if FF_Flag
        Vel_FF = single(-Stewart_Heave_Vel);
    else
        Vel_FF = single(0);
    end

== matlab function sg_IK/Controller/Winch_Controller/Winch_StewartFB_Based_HeaveComp/If_EndEff_OverPlatform ==
  data: FK_Pos input; IsWithin output
function IsWithin = OverEM1500(FK_Pos)
    %checks if the x and y coordinate of the robot end effector is withing
    %the coordinates of the stewart platfrom em1500
    x = FK_Pos(1); y = FK_Pos(2);
    cx = 3.17;         cy = 0.24;
    r = 0.85;

    % Calculate the squared distance from the point (x,y) to the center (cx,cy)
    distSq = (x - cx)^2 + (y - cy)^2;

    % Calculate the squared radius
    radiusSq = r^2;

    % Check if the point's squared distance is less than or equal to the squared radius
    % Using squared values avoids using sqrt(), which is computationally cheaper.
    if distSq <= radiusSq
        IsWithin = 1; % Point is inside or on the boundary
    else
        IsWithin = 0; % Point is outside
    end

end

== matlab function sg_IK/Controller/Winch_Controller/Winch_Camera_Based_HeaveComp/Winch_Local_to_Global ==
  data: FK_Pos input; Winch_Global_Pos_Z output; Winch_Length input
function Winch_Global_Pos_Z = Winch_Global_Pos(FK_Pos, Winch_Length)

    % Calculate actual vertical distance below end-effector
    vertical_distance = Winch_Length - 0.202; 

    % Calculate hook global position [X, Y, Z]
    Winch_Global_Pos_Z = FK_Pos(3) - vertical_distance;

end

== matlab function sg_IK/Controller/Winch_Controller/Winch_StewartFB_Based_HeaveComp/Winch_Posref_ramp_generator ==
  data: new_command input; Winch_PosRef_Input input; Winch_Pos input; PosRef output; t input; Vel_FF output; Em1500_Heave input; Em1500_Heave_Vel input; Enable_HeaveComp input
function [PosRef, Vel_FF] = WinchTrajectory(new_command, Winch_PosRef_Input, Winch_Pos, t, Em1500_Heave, Em1500_Heave_Vel, Enable_HeaveComp)

Em1500_Heave       = Em1500_Heave;
Em1500_Heave_Vel   = Em1500_Heave_Vel; % CHECK SIGN
%Em1500_Heave_world = -Em1500_Heave + 1.886;

%Flag for if platform is in settled position
%Better handling would be a direct feedback from the Em1500 IPC what operation mode the platform is in
if Em1500_Heave >= 0.464 && Em1500_Heave <= 0.468 %Em1500 platform is in settled mode
    Em1500_Settled_Flag = true;
else
    Em1500_Settled_Flag = false;
end

v_command_speed = 0.05; %Low speed to lower payload carefully


%Persistent variables
persistent last_command is_moving command_start_time command_start_pos current_target_pos T_move actual_move_vel
persistent target_idle_base_pos
persistent first_run


if isempty(first_run)
    last_command = new_command;
    is_moving = false;
    command_start_time = t;
    T_move = 0;
    actual_move_vel = 0;
    
    target_idle_base_pos = Winch_Pos; 
    command_start_pos = target_idle_base_pos; 
    current_target_pos = target_idle_base_pos;


    first_run = false;
end


%Detect new command then plan ramp 
if new_command ~= last_command
    command_start_pos = Winch_Pos; % Start ramp from last base position
    current_target_pos = Winch_PosRef_Input;
    delta_pos = current_target_pos - command_start_pos;


    %Check if a move is needed and possible
    if abs(delta_pos) > 1e-6
        is_moving = true;
        command_start_time = t;
        direction = sign(delta_pos);%Find sign of direction move
        actual_move_vel = direction * v_command_speed;
        T_move = abs(delta_pos) / v_command_speed;
    else
        %No move needed winch is allready at target position
        is_moving = false;
        T_move = 0;
        actual_move_vel = 0;

        if abs(delta_pos) <= 1e-6
             target_idle_base_pos = current_target_pos;
        end
    end
    last_command = new_command;
end


%Commanded Position and Velocity 
Commanded_Pos = target_idle_base_pos; %Default to base position
Commanded_Vel = 0; %Default to zero velocity without heave comp


if is_moving
    local_t = t - command_start_time;


    if local_t < T_move && T_move > 0
        %Ramp in progress
        Commanded_Pos = command_start_pos + actual_move_vel * local_t;
        Commanded_Vel = actual_move_vel;
    else
        %Ramp finished
        Commanded_Pos = current_target_pos;
        Commanded_Vel = 0;
        target_idle_base_pos = current_target_pos; %Update base position
        is_moving = false; %Stop the move state
        actual_move_vel = 0; %Reset velocity
        T_move = 0; %Reset duration
    end
end

%Heave compensation
if Enable_HeaveComp && ~Em1500_Settled_Flag
    %Heave compensation activated
    PosRef = Commanded_Pos - Em1500_Heave;
    %PosRef = Commanded_Pos;
    Vel_FF = Commanded_Vel - Em1500_Heave_Vel; %Feedforward vel for controller
else
    PosRef = Commanded_Pos;
    Vel_FF = Commanded_Vel;
end


end
